simulink library "ScaleOneEighty"  (R2020a)
settings: Solver=VariableStepAuto  StartTime=0.0  StopTime=10.0  RelTol=1e-3
settings Model: Creator=marqu  LastModifiedBy=marqu

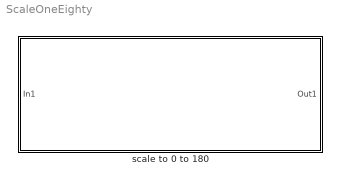
== system ScaleOneEighty ==
  scale to 0 to 180 : Subsystem

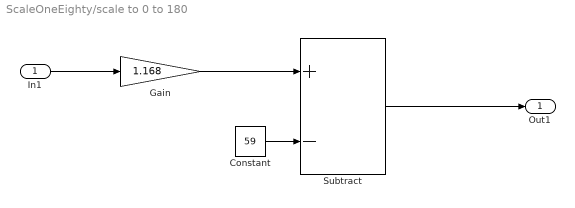
== system ScaleOneEighty/scale to 0 to 180 ==
  In1 : Inport
  Constant : Constant  Value=59  OutDataTypeStr=uint8
  Gain : Gain  Gain=1.168  OutDataTypeStr=single
  Subtract : Sum  Inputs=+-  OutDataTypeStr=uint8
  Out1 : Outport
  wires:
  Constant/1 -> Subtract/2
  Gain/1 -> Subtract/1
  Subtract/1 -> Out1/1
  In1/1 -> Gain/1
